simulink model "ex_massa_molla_smorzatore"  (R2024b)
settings: Solver=VariableStepAuto  StartTime=0.0  StopTime=60  RelTol=1e-3

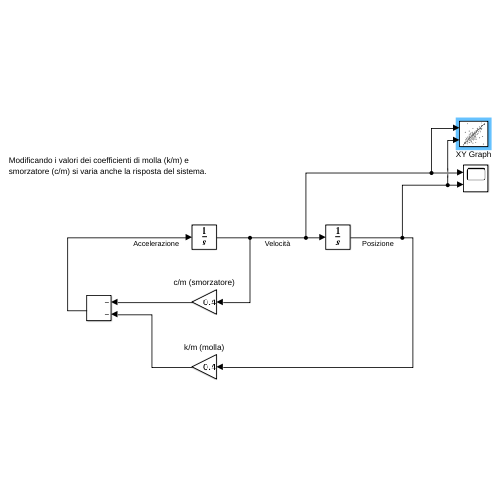
[thumbnail: Simulink's stored preview of the top-level diagram]
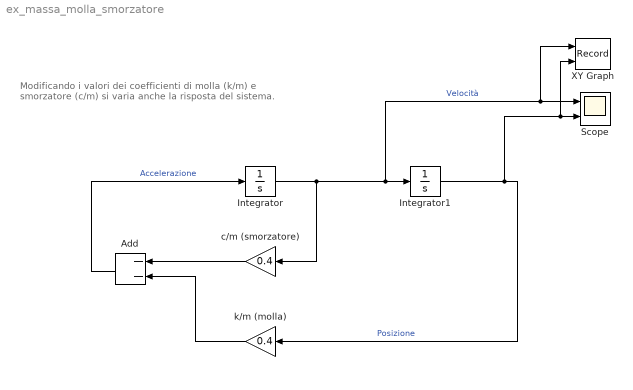
== system ex_massa_molla_smorzatore ==
  note: Modificando i valori dei coefficienti di molla (k/m) e
      | smorzatore (c/m) si varia anche la risposta del sistema.
  Add : Sum  Inputs=--
  Integrator : Integrator
  Integrator1 : Integrator  InitialCondition=1
  Scope : Scope  NumInputPorts=2
  XY Graph : Record  FileSettingsInternal="{\"entries\":[{\"content\":{\"excelSettings\":{\"content\":{},\"type\":\"Streamout.ExcelSettings\"}},\"type\":\"Streamout.FileSettingStorage\",\"uuid\":\"\"}],\"packageUris\":[\"http:\\/\\/schema.mathworks.com\\/mf0\\/streamout_blocks\\/R2020a\"],\"version\":\"1.0\"}"  Layout=OverlayBottom  SignalsInternal="{\"entries\":[{\"content\":{\"signals\":[{\"content\":{\"blockPath\":[],\"dimensions\":[1],\"domain\":\"\",\"lineColor\":\"#a2142f\",\"plots\":[ 1, 2 ],\"port\":1,\"sid\":[\"\"],\"signalID\":1,\"signalName\":\"Velocità\"},\"type\":\"RecordBlkView.Signal\",\"uuid\":\"\"},{\"content\":{\"blockPath\":[],\"dimensions\":[1],\"domain\":\"\",\"lineColor\":\"#139fff\",\"plots\":[ 1, 9 ],\"port\":2,\"sid\":[\"\"],\"signalID\":2,\"signalName\":\"Posizione\"},\"type\":\"RecordBlkView.Signal\",\"uuid\":\"\"}]},\"type\":\"RecordBlkView.InputSignals\",\"uuid\":\"\"}],\"packageUris\":[\"http:\\/\\/schema.mathworks.com\\/mf0\\/streamout_blocks\\/R2020a\"],\"version\":\"1.0\"}"  VisualizationBindings="{\"sparklinesplugin\":{\"info\":[{\"bindingParametersList\":[],\"subplotID\":2}]},\"xyplotplugin\":{\"info\":[{\"series\":[{\"bindingParametersList\":[{\"parameter\":\"X-Axis\",\"signalID\":1,\"signalName\":\"Velocità\"},{\"parameter\":\"Y-Axis\",\"signalID\":2,\"signalName\":\"Posizione\"},{\"parameter\":\"X-Axis\",\"signalID\":1,\"signalName\":\"Velocità\"},{\"parameter\":\"Y-Axis\",\"signalID\":2,\"signalName\":\"Posizione\"}],\"seriesID\":0}],\"subplotID\":1}]}}"  CompatibilityTag=XY
  c/m (smorzatore) : Gain  Gain=0.4
  k/m (molla) : Gain  Gain=0.4
  wires:
  Integrator/1 -> c/m (smorzatore)/1, XY Graph/1, Scope/1, Integrator1/1  "Velocità"
  Add/1 -> Integrator/1  "Accelerazione"
  Integrator1/1 -> XY Graph/2, Scope/2, k/m (molla)/1  "Posizione"
  c/m (smorzatore)/1 -> Add/1
  k/m (molla)/1 -> Add/2
